simulink model "complete_model_sim_nolib"  (R2023b)
settings: Solver=VariableStepAuto  StartTime=0.0  StopTime=1e4  RelTol=1e-3
values from neighbouring files (symbols this model uses):
  a = 6.851221970532768e+03    (= 6851.22197053)    [complete_model.m]
  alpha1 = 0.4    [complete_model.m]
  alpha2 = 0.1    [complete_model.m]
  alpha3 = 0.5    [complete_model.m]
  D = zeros(3)    [complete_model.m]
  e = 0    [complete_model.m]
  FOV_earth = deg2rad(33)    [complete_model.m]
  FOV_sun = deg2rad(100)    [complete_model.m]
  freq_earth = 5    [complete_model.m]
  freq_mag = 5    [complete_model.m]
  freq_sun = 5    [complete_model.m]
  I = diag([I1 I2 I3])    [complete_model.m]    (also in compute_integral.m = I + (y(i + 1) + y(i) ) * (t(i + 1) - t(i)) * 0.5)
  Iinv = I\eye(3)    [complete_model.m]
  jb = [0.01; 0.05; 0.01]    [complete_model.m]
  k_gain = (4*pi/T) * (1 + sin(chsi)) * I2    [complete_model.m]
  mu = astroConstants(13)    [complete_model.m]
  n = sqrt(mu/a^3)    [complete_model.m]
  omega0 = 0.06 * rand(3,1)    [complete_model.m]
  omegaE = deg2rad(15)/3600    [complete_model.m]
  rs = -rr    [complete_model.m]
  s0 = 2*pi*rand(3,1)    [complete_model.m]
  tol = 0.2    [complete_model.m]
undefined symbols (not defined in the file or in its folder): gh, magnitude
libraries: cstextras x3, matrix_library x2, simulink_extras x1
(part 1 of 3)
settings Model: Creator=marcellopareschi  LastModifiedBy=turcu

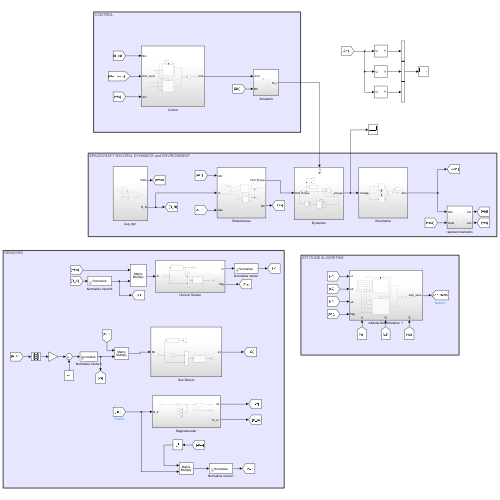
[thumbnail: Simulink's stored preview of the top-level diagram]
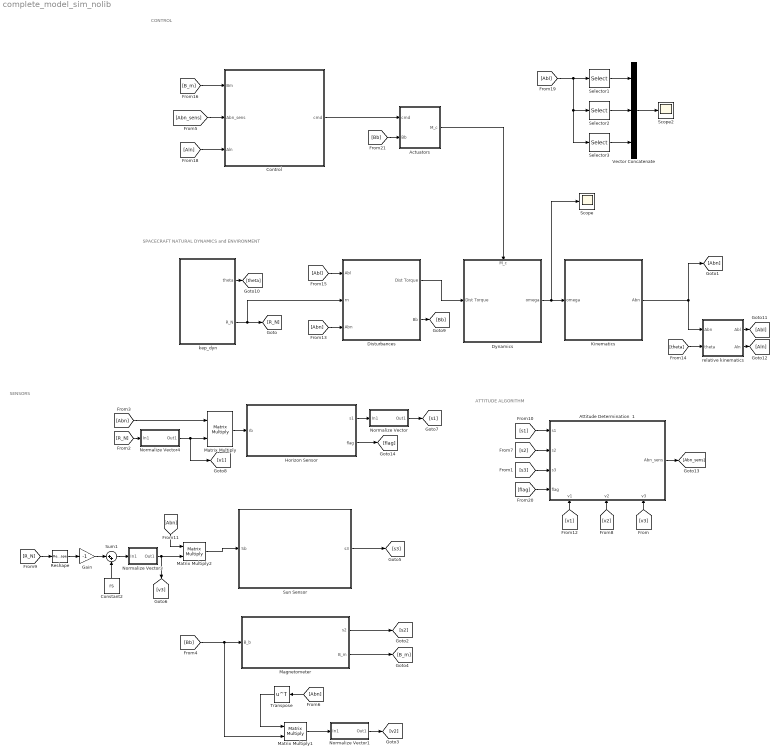
== system complete_model_sim_nolib ==
  note: SPACECRAFT NATURAL DYNAMICS and ENVIRONMENT
  note: CONTROL
  note: ATTITUDE ALGORITHM
  note: SENSORS
  " Actuators" : Subsystem
  Attitude Determination  1 : Subsystem
      settings: PortSchema="{\"entries\":[{\"content\":{\"sides\":[{\"content\":{\"connectorIds\":[\"In1\",\"In2\",\"In3\",\"In4\"]},\"type\":\"ConnectorPlacement.EquallySpacedRectSide\",\"uuid\":\"730966cf-d0d7-44a0-92f0-b5324480e7cc\"},{\"content\":{\"connectorIds\":[\"Out1\"],\"side\":\"RIGHT\"},\"type\":\"ConnectorPlacement.EquallySpacedRectSide\",\"uuid\":\"c83e6b57-46fe-4a45-9824-d3495e15bf6a\"},{\"content\":{\"side\":\"TOP\"},\"type\":\"ConnectorPlacement.EquallySpacedRectSide\",\"uuid\":\"4938c298-c2b3-45b7-bcb0-70b8132dabc6\"},{\"content\":{\"connectorIds\":[\"In5\",\"In6\",\"In7\"],\"side\":\"BOTTOM\"},\"type\":\"ConnectorPlacement.EquallySpacedRectSide\",\"uuid\":\"6d6a244e-80db-423b-a0a5-9a5face48fcb\"}]},\"type\":\"ConnectorPlacement.EquallySpacedConnector\",\"uuid\":\"7eb6767d-3ff0-4577-86c9-ebc5e763f220\"}],\"packageUris\":[\"http://schema.mathworks.com/mf0/Connector/R2020b\"],\"version\":\"1.0\"}"
  Constant2 : Constant  Value=rs
  Control : Subsystem
  Disturbances : Subsystem
  Dynamics : Subsystem
      settings: PortSchema="{\"entries\":[{\"content\":{\"sides\":[{\"content\":{\"connectorIds\":[\"In1\"]},\"type\":\"ConnectorPlacement.EquallySpacedRectSide\",\"uuid\":\"c50eaaef-bc5a-4b30-975a-dad3b72c53e1\"},{\"content\":{\"connectorIds\":[\"Out1\"],\"side\":\"RIGHT\"},\"type\":\"ConnectorPlacement.EquallySpacedRectSide\",\"uuid\":\"08d23e91-5daf-4f03-95f9-71d6696597c3\"},{\"content\":{\"connectorIds\":[\"In2\"],\"side\":\"TOP\"},\"type\":\"ConnectorPlacement.EquallySpacedRectSide\",\"uuid\":\"7ec65280-cc3e-44b1-8843-81c3a216d755\"}]},\"type\":\"ConnectorPlacement.EquallySpacedConnector\",\"uuid\":\"721d018a-ab6c-4a15-8dbf-409a72b03ba1\"}],\"packageUris\":[\"http://schema.mathworks.com/mf0/Connector/R2020b\"],\"version\":\"1.0\"}"
  Gain : Gain  Gain=-1
  Horizon Sensor : Subsystem
  Kinematics : Subsystem
  Magnetometer : Subsystem
  Matrix Multiply : Product  Multiplication=Matrix(*)
  Matrix Multiply1 : Product  Multiplication=Matrix(*)
  Matrix Multiply2 : Product  Multiplication=Matrix(*)
  Normalize Vector : Subsystem  mask(Normalize Vector){maxzero=0}
      mask prompts: maxzero "Maximum modulus to treat vector as zero:"
      mask help:
      | Normalize a vector.
      | Output is the unit vector parallel to the input vector. Input can be vector of any size.
      | If the modulus of the input is lower or equal than specified, the output is set to zeros(size(u)).
      settings: LibrarySourceBlock=vrlib/Utilities/Normalize Vector
      mask Help: helpview(vrmfunc('FnHelpTopic'), 'vr_normalizevector');
      mask Display: disp('Normalize')
  Normalize Vector1 : Subsystem  mask(Normalize Vector){maxzero=0}
      mask prompts: maxzero "Maximum modulus to treat vector as zero:"
      mask help:
      | Normalize a vector.
      | Output is the unit vector parallel to the input vector. Input can be vector of any size.
      | If the modulus of the input is lower or equal than specified, the output is set to zeros(size(u)).
      settings: LibrarySourceBlock=vrlib/Utilities/Normalize Vector
      mask Help: helpview(vrmfunc('FnHelpTopic'), 'vr_normalizevector');
      mask Display: disp('Normalize')
  Normalize Vector3 : Subsystem  mask(Normalize Vector){maxzero=0}
      mask prompts: maxzero "Maximum modulus to treat vector as zero:"
      mask help:
      | Normalize a vector.
      | Output is the unit vector parallel to the input vector. Input can be vector of any size.
      | If the modulus of the input is lower or equal than specified, the output is set to zeros(size(u)).
      settings: LibrarySourceBlock=vrlib/Utilities/Normalize Vector
      mask Help: helpview(vrmfunc('FnHelpTopic'), 'vr_normalizevector');
      mask Display: disp('Normalize')
  Normalize Vector4 : Subsystem  mask(Normalize Vector){maxzero=0}
      mask prompts: maxzero "Maximum modulus to treat vector as zero:"
      mask help:
      | Normalize a vector.
      | Output is the unit vector parallel to the input vector. Input can be vector of any size.
      | If the modulus of the input is lower or equal than specified, the output is set to zeros(size(u)).
      settings: LibrarySourceBlock=vrlib/Utilities/Normalize Vector
      mask Help: helpview(vrmfunc('FnHelpTopic'), 'vr_normalizevector');
      mask Display: disp('Normalize')
  Reshape : Reshape  OutputDimensionality=Column vector (2-D)
  Scope : Scope
  Scope2 : Scope
  Selector1 : Selector  NumberOfDimensions=2  InputPortWidth=3  IndexOptions=Index vector (dialog),Index vector (dialog)  Indices=3,2  OutputSizes=1,1
  Selector2 : Selector  NumberOfDimensions=2  InputPortWidth=3  IndexOptions=Index vector (dialog),Index vector (dialog)  Indices=1,3  OutputSizes=1,1
  Selector3 : Selector  NumberOfDimensions=2  InputPortWidth=3  IndexOptions=Index vector (dialog),Index vector (dialog)  Indices=2,1  OutputSizes=1,1
  Sum1 : Sum  Inputs=|++
  Sun Sensor : Subsystem
  Transpose : Math  Operator=transpose
  Vector Concatenate : Concatenate  NumInputs=3
  kep_dyn : Subsystem
  relative kinematics : Subsystem
  wires:
  Normalize Vector3/1(Out1) -> Matrix Multiply2/2, [v3]
  Magnetometer/1(s2) -> [s2]
  [Abn] -> Transpose/1
  Matrix Multiply1/1 -> Normalize Vector1/1(In1)
  Transpose/1 -> Matrix Multiply1/1
  [theta] -> relative kinematics/2(theta)
  [v1] -> Attitude Determination  1/5(v1)
  [Abn] -> Matrix Multiply/1
  [R_N] -> Reshape/1
  Gain/1 -> Sum1/1
  [Bb] -> Matrix Multiply1/2, Magnetometer/1(B_b)
  Normalize Vector4/1(Out1) -> [v1], Matrix Multiply/2
  [s3] -> Attitude Determination  1/3(s3)
  Normalize Vector1/1(Out1) -> [v2]
  " Actuators"/1(M_c) -> Dynamics/2(M_c)
  Magnetometer/2("B_m ") -> [B_m]
  Sun Sensor/1(s3) -> [s3]
  [R_N] -> Normalize Vector4/1(In1)
  Constant2/1 -> Sum1/2
  [s2] -> Attitude Determination  1/2(s2)
  Matrix Multiply/1 -> Horizon Sensor/1(rb)
  Reshape/1 -> Gain/1
  Normalize Vector/1(Out1) -> [s1]
  [v3] -> Attitude Determination  1/7(v3)
  [s1] -> Attitude Determination  1/1(s1)
  Sum1/1 -> Normalize Vector3/1(In1)
  Attitude Determination  1/1(Abn_sens) -> [Abn_sens]
  relative kinematics/1(Abl) -> [Abl]
  Kinematics/1(Abn) -> [Abn], relative kinematics/1(Abn)
  relative kinematics/2(Aln) -> [Aln]
  [Abn] -> Matrix Multiply2/1
  Dynamics/1(omega) -> Scope/1, Kinematics/1(omega)
  [v2] -> Attitude Determination  1/6(v2)
  Horizon Sensor/1(s1) -> Normalize Vector/1(In1)
  Matrix Multiply2/1 -> Sun Sensor/1(Sb)
  [Bb] -> " Actuators"/2(Bb)
  [B_m] -> Control/1(Bm)
  [Abn_sens] -> Control/2(Abn_sens)
  [Aln] -> Control/3(Aln)
  Control/1(cmd) -> " Actuators"/1(cmd)
  [Abl] -> Selector3/1, Selector2/1, Selector1/1
  Selector2/1 -> Vector Concatenate/2
  Selector3/1 -> Vector Concatenate/3
  Selector1/1 -> Vector Concatenate/1
  Vector Concatenate/1 -> Scope2/1
  Horizon Sensor/2(flag) -> [flag]
  [flag] -> Attitude Determination  1/4(flag)
  [Abl] -> Disturbances/1(Abl)
  kep_dyn/1(theta) -> [theta]
  [Abn] -> Disturbances/3(Abn)
  Disturbances/1(Dist Torque) -> Dynamics/1(Dist Torque)
  Disturbances/2(Bb) -> [Bb]
  kep_dyn/2(R_N) -> Disturbances/2(rn), [R_N]

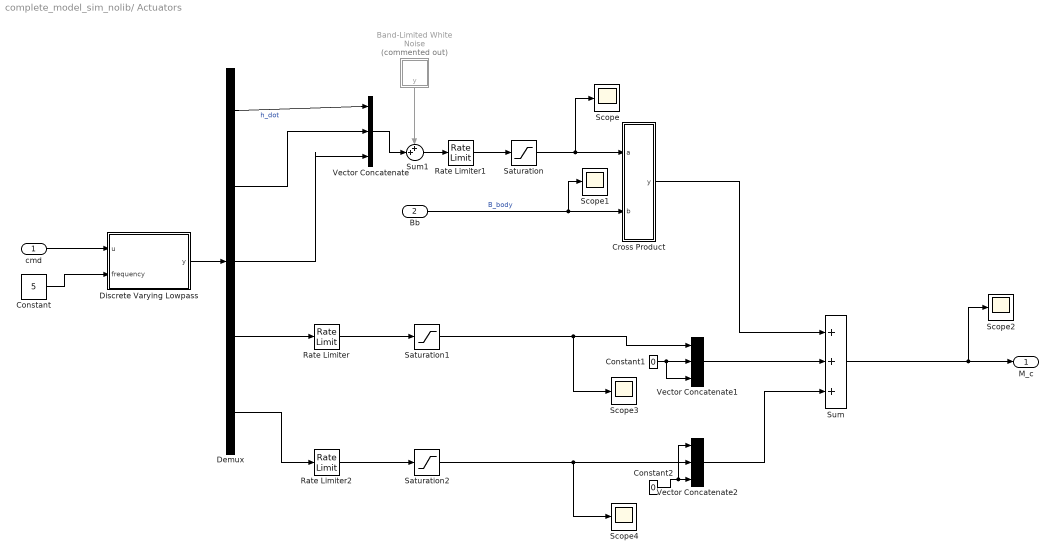
== system complete_model_sim_nolib/ Actuators ==
  cmd : Inport
  Bb : Inport  Port=2
  Band-Limited White Noise : Subsystem  Commented=on  mask(Band-Limited White Noise.){Cov=[0.1], Ts=1/30, seed=[23341], VectorParams1D=on}
      mask prompts: Cov "Simulink:masks:NoisePower_MP"; Ts "Simulink:masks:SampleTime_MP"; seed "Simulink:masks:Seed_MP"; VectorParams1D "Simulink:masks:InterpretVectorParametersAs1D_MP"
      mask help: Simulink:masks:BandLimitedWhiteNoise_MD
      mask init:
      | if any(Cov < 0),
      | 	error('The ''Noise power'' must be positive. '),
      | end;
      | 
      | r = [-0.4326
      |    -1.6656
      |     0.1253
      |     0.2877
      |    -1.1465
      |     1.1909
      |     1.1892
      |    -0.0376
      |     0.3273
      |     0.1746
      |    -0.1867
      |     0.7258]';
      | 
      | r2 = [r(1),r;r,r(12)]; 
      | t =[1:13;1:13]; 
      | 
      | if any(Ts==-1), 
      | 	error('Sample time (-1) is set to be back-inherited from the block(s) it drives. You should explicitly specify the sample time of the source block. '), 
      | end;
      | 
      | if ~isdeployed
      | set_param([gcb '/White Noise'],'VectorParams1D',VectorParams1D);
      | end
      settings: LibrarySourceBlock=|
      | simulink/Sources/Band-Limited
      | White Noise
      mask Help: Implemented using white noise into Zero-Order Hold block. The seed and power can be vectors of the same length to produce a vector of white noise sources. For faster simulation, set sample time to the highest value possible but in accordance with the fastest dynamics of system.
  Constant : Constant  Value=5
  Constant1 : Constant  Value=0
  Constant2 : Constant  Value=0
  Cross Product : Subsystem  mask(CrossProduct){}
      mask help: Simulink:masks:MatLibCrossProduct_MD
      settings: LibrarySourceBlock=|
      | simulink/Matrix
      | Operations/Cross Product
      mask Display: disp('cross')
  Demux : Demux  Outputs=5
  Discrete Varying Lowpass : Subsystem  mask(Discrete Varying Lowpass){N=2, w0=0, Ts=1/30}
      mask prompts: N "Control:simulink:VaryingLowpassLabel1"; w0 "Control:simulink:VaryingLowpassLabel2"; Ts "Control:simulink:VaryingLowpassLabel3"
      mask help: Control:simulink:VaryingLowpass2
      mask init:
      | if N~=round(N)
      |    hCB = get_param(gcb,'handle');
      |    DAStudio.slerror('Control:simulink:InvalidOrder',hCB)
      | elseif w0*Ts>=pi
      |    hCB = get_param(gcb,'handle');
      |    DAStudio.slerror('Control:simulink:InvalidPrewarp',hCB)
      | end
      | SimStatus = get_param(bdroot,'SimulationStatus');
      | if any(strcmp(SimStatus,{'initializing','updating','stopped'}))
      |    controllib.internal.blocks.varying.varyingLP(gcb,N,Ts)
      | end
      settings: LibrarySourceBlock=cstblocks/Linear Parameter Varying/Discrete Varying Lowpass
      mask Help: eval('helpview(''control'',''VaryingLowpassDT'');')
      mask DialogControl N Prompt: Filter order:
      mask DialogControl w0 Prompt: Pre-warping frequency w0 (rad/s):
      mask DialogControl Ts Prompt: Sample time Ts:
      mask Display:
      | image('lowpass_dt.png',[0.1 0 0.8 1]);
      | port_label('input', 2, 'freq');
  Rate Limiter : RateLimiter
  Rate Limiter1 : RateLimiter  RisingSlewLimit=10  FallingSlewLimit=-10
  Rate Limiter2 : RateLimiter
  Saturation : Saturate  UpperLimit=150  LowerLimit=-150
  Saturation1 : Saturate
  Saturation2 : Saturate
  Scope{,1..4} (5 alike) : Scope
  Sum : Sum  Inputs=+++
  Sum1 : Sum  Inputs=++|
  Vector Concatenate : Concatenate  NumInputs=3
  Vector Concatenate1 : Concatenate  NumInputs=3
  Vector Concatenate2 : Concatenate  NumInputs=3
  M_c : Outport
  wires:
  Bb/1 -> Scope1/1, Cross Product/2(b)  "B_body"
  Rate Limiter1/1 -> Saturation/1
  Band-Limited White Noise/1(y) -> Sum1/1
  Sum1/1 -> Rate Limiter1/1
  Saturation/1 -> Scope/1, Cross Product/1(a)
  Vector Concatenate/1 -> Sum1/2
  Constant1/1 -> Vector Concatenate1/3, Vector Concatenate1/2
  Sum/1 -> Scope2/1, M_c/1
  Rate Limiter/1 -> Saturation1/1
  Saturation1/1 -> Scope3/1, Vector Concatenate1/1
  Demux/1 -> Vector Concatenate/1  "h_dot"
  Demux/2 -> Vector Concatenate/2
  Demux/3 -> Vector Concatenate/3
  Demux/4 -> Rate Limiter/1
  Saturation2/1 -> Vector Concatenate2/2, Scope4/1
  Constant2/1 -> Vector Concatenate2/1, Vector Concatenate2/3
  Rate Limiter2/1 -> Saturation2/1
  Demux/5 -> Rate Limiter2/1
  Vector Concatenate1/1 -> Sum/2
  Cross Product/1(y) -> Sum/1
  Vector Concatenate2/1 -> Sum/3
  Constant/1 -> Discrete Varying Lowpass/2(frequency)
  Discrete Varying Lowpass/1(y) -> Demux/1
  cmd/1 -> Discrete Varying Lowpass/1(u)

== system complete_model_sim_nolib/Attitude Determination  1 ==
  s1 : Inport
  s2 : Inport  Port=2
  s3 : Inport  Port=3
  flag : Inport  Port=4
  v1 : Inport  Port=5
  v2 : Inport  Port=6
  v3 : Inport  Port=7
  Enabled Subsystem : Subsystem  TreatAsAtomicUnit=on
  Merge : Merge
  NOT : Logic  Operator=NOT  IconShape=distinctive  AllPortsSameDT=off  OutDataTypeStr=boolean
  Statistical Method : Subsystem  TreatAsAtomicUnit=on
  Abn_sens : Outport
  wires:
  flag/1 -> NOT/1, Statistical Method/Enable
  s1/1 -> Statistical Method/1(s1)
  s2/1 -> Enabled Subsystem/1(q), Statistical Method/2(s2)
  s3/1 -> Enabled Subsystem/2(p), Statistical Method/3(s3)
  v1/1 -> Statistical Method/4(v1)
  v2/1 -> Enabled Subsystem/3(b), Statistical Method/5(v2)
  v3/1 -> Enabled Subsystem/4(a), Statistical Method/6(v3)
  NOT/1 -> Enabled Subsystem/Enable
  Statistical Method/1(Abn_sens) -> Merge/1
  Enabled Subsystem/1(A_bn_sens) -> Merge/2
  Merge/1 -> Abn_sens/1

== system complete_model_sim_nolib/Control ==
  Bm : Inport
  Abn_sens : Inport  Port=2
  Aln : Inport  Port=3
  De-Tumbling Bdot control1 : Subsystem
  Merge : Merge
  NOT : Logic  Operator=NOT  IconShape=distinctive  AllPortsSameDT=off  OutDataTypeStr=boolean
  Scope1 : Scope
  Slew Maneuver : Subsystem
  Unit Delay : UnitDelay  InitialCondition=1  SampleTime=-1  HasFrameUpgradeWarning=on
  cmd : Outport
  wires:
  Unit Delay/1 -> NOT/1, Scope1/1, De-Tumbling Bdot control1/Enable
  De-Tumbling Bdot control1/2(flag) -> Unit Delay/1
  Bm/1 -> Slew Maneuver/3(B_m), De-Tumbling Bdot control1/1(B_m)
  Abn_sens/1 -> Slew Maneuver/1(Abn_sens)
  Aln/1 -> Slew Maneuver/2(Aln)
  NOT/1 -> Slew Maneuver/Enable
  Slew Maneuver/1(cmd) -> Merge/2
  De-Tumbling Bdot control1/1(cmd) -> Merge/1
  Merge/1 -> cmd/1

== system complete_model_sim_nolib/Disturbances ==
  Abl : Inport
  rn : Inport  Port=2
  Abn : Inport  Port=3
  Constant : Constant  Value=[1; 0; 0]
  "Magnetic Torque " : Subsystem
  Matrix Multiply : Product  Multiplication=Matrix(*)
  Scope1 : Scope
  Sum : Sum  Inputs=|++
  To Workspace : ToWorkspace  VariableName=GG_torque  SampleTime=-1
  To Workspace1 : ToWorkspace  VariableName=mag_torque  SampleTime=-1
  gravity torque : Subsystem
  norm : Subsystem
  Dist Torque : Outport
  Bb : Outport  Port=2
  wires:
  Abl/1 -> Matrix Multiply/1
  Constant/1 -> Matrix Multiply/2
  Matrix Multiply/1 -> gravity torque/1(c)
  rn/1 -> norm/1(rn), "Magnetic Torque "/1(rn)
  Abn/1 -> "Magnetic Torque "/2(Abn)
  gravity torque/1(Mg) -> To Workspace/1, Sum/1
  "Magnetic Torque "/1(M_mag) -> To Workspace1/1, Sum/2, Scope1/1
  Sum/1 -> Dist Torque/1
  "Magnetic Torque "/2(Bb) -> Bb/1
  norm/1(rnorm) -> gravity torque/2(rnorm)

== system complete_model_sim_nolib/Dynamics ==
  Dist Torque : Inport
  M_c : Inport  Port=2
  Constant : Constant  Value=I
  Constant1 : Constant  Value=Iinv
  Cross Product : Subsystem  mask(CrossProduct){}
      mask help: Simulink:masks:MatLibCrossProduct_MD
      settings: LibrarySourceBlock=|
      | simulink/Matrix
      | Operations/Cross Product
      mask Display: disp('cross')
  Integrator : Integrator  InitialCondition=omega0
  Product : Product  Multiplication=Matrix(*)
  Product1 : Product  Multiplication=Matrix(*)
  Scope : Scope
  Scope1 : Scope
  Sum : Sum  Inputs=+++
  To Workspace : ToWorkspace  VariableName=omegab  SampleTime=-1
  omega : Outport
  wires:
  Constant/1 -> Product/1
  Product1/1 -> Integrator/1
  Integrator/1 -> omega/1, Scope/1, To Workspace/1, Cross Product/2(b), Product/2
  Product/1 -> Cross Product/1(a)
  Constant1/1 -> Product1/1
  Cross Product/1(y) -> Sum/2
  Sum/1 -> Product1/2
  Dist Torque/1 -> Sum/3
  M_c/1 -> Scope1/1, Sum/1

== system complete_model_sim_nolib/Horizon Sensor ==
  rb : Inport
  EH sensor modeling : Subsystem
  FOV CHECK : Subsystem
  Product1 : Product
  s1 : Outport
  flag : Outport  Port=2
  wires:
  rb/1 -> FOV CHECK/1(rb), Product1/2
  Product1/1 -> EH sensor modeling/1(rb)
  EH sensor modeling/1(q) -> s1/1  "direction of earth"
  FOV CHECK/1(b) -> Product1/1, flag/1

== system complete_model_sim_nolib/Kinematics ==
  omega : Inport
  Kinematics 312 : Subsystem
  Kinematics 313 : Subsystem
  Merge : Merge
  NOT : Logic  Operator=NOT  IconShape=distinctive  AllPortsSameDT=off  OutDataTypeStr=boolean
  System switcher : Subsystem
  To Workspace : ToWorkspace  VariableName=A  SaveFormat=Timeseries  SampleTime=-1
  Abn : Outport
  wires:
  NOT/1 -> Kinematics 313/Enable
  omega/1 -> Kinematics 312/1(w), Kinematics 313/1(w)
  System switcher/1(flag) -> Kinematics 312/Enable, NOT/1
  Kinematics 313/1(A) -> Merge/2
  Merge/1 -> Abn/1, To Workspace/1  "A"
  Kinematics 312/1(A) -> Merge/1

== system complete_model_sim_nolib/Magnetometer ==
  B_b : Inport
  Band-Limited White Noise : Subsystem  mask(Band-Limited White Noise.){Cov=[1.18^2 *1e-18], Ts=1/30, seed=[23341], VectorParams1D=on}
      mask prompts: Cov "Simulink:masks:NoisePower_MP"; Ts "Simulink:masks:SampleTime_MP"; seed "Simulink:masks:Seed_MP"; VectorParams1D "Simulink:masks:InterpretVectorParametersAs1D_MP"
      mask help: Simulink:masks:BandLimitedWhiteNoise_MD
      mask init: same as complete_model_sim_nolib/ Actuators/Band-Limited White Noise
      settings: LibrarySourceBlock=|
      | simulink/Sources/Band-Limited
      | White Noise
      mask Help: Implemented using white noise into Zero-Order Hold block. The seed and power can be vectors of the same length to produce a vector of white noise sources. For faster simulation, set sample time to the highest value possible but in accordance with the fastest dynamics of system.
  Band-Limited White Noise1 : Subsystem  mask(Band-Limited White Noise.){Cov=[1.18^2 *1e-18], Ts=1/30, seed=[23341], VectorParams1D=on}
      mask prompts: Cov "Simulink:masks:NoisePower_MP"; Ts "Simulink:masks:SampleTime_MP"; seed "Simulink:masks:Seed_MP"; VectorParams1D "Simulink:masks:InterpretVectorParametersAs1D_MP"
      mask help: Simulink:masks:BandLimitedWhiteNoise_MD
      mask init: same as complete_model_sim_nolib/ Actuators/Band-Limited White Noise
      settings: LibrarySourceBlock=|
      | simulink/Sources/Band-Limited
      | White Noise
      mask Help: Implemented using white noise into Zero-Order Hold block. The seed and power can be vectors of the same length to produce a vector of white noise sources. For faster simulation, set sample time to the highest value possible but in accordance with the fastest dynamics of system.
  Band-Limited White Noise2 : Subsystem  mask(Band-Limited White Noise.){Cov=[1.18^2 *1e-18], Ts=1/30, seed=[23341], VectorParams1D=on}
      mask prompts: Cov "Simulink:masks:NoisePower_MP"; Ts "Simulink:masks:SampleTime_MP"; seed "Simulink:masks:Seed_MP"; VectorParams1D "Simulink:masks:InterpretVectorParametersAs1D_MP"
      mask help: Simulink:masks:BandLimitedWhiteNoise_MD
      mask init: same as complete_model_sim_nolib/ Actuators/Band-Limited White Noise
      settings: LibrarySourceBlock=|
      | simulink/Sources/Band-Limited
      | White Noise
      mask Help: Implemented using white noise into Zero-Order Hold block. The seed and power can be vectors of the same length to produce a vector of white noise sources. For faster simulation, set sample time to the highest value possible but in accordance with the fastest dynamics of system.
  Normalize Vector : Subsystem  mask(Normalize Vector){maxzero=0}
      mask prompts: maxzero "Maximum modulus to treat vector as zero:"
      mask help:
      | Normalize a vector.
      | Output is the unit vector parallel to the input vector. Input can be vector of any size.
      | If the modulus of the input is lower or equal than specified, the output is set to zeros(size(u)).
      settings: LibrarySourceBlock=vrlib/Utilities/Normalize Vector
      mask Help: helpview(vrmfunc('FnHelpTopic'), 'vr_normalizevector');
      mask Display: disp('Normalize')
  Sum : Sum  Inputs=|++
  Vector Concatenate1 : Concatenate  NumInputs=3
  Zero-Order Hold2 : ZeroOrderHold  SampleTime=1/freq_mag
  s2 : Outport
  "B_m " : Outport  Port=2
  wires:
  Zero-Order Hold2/1 -> Sum/1  "B_B"
  Band-Limited White Noise2/1(y) -> Vector Concatenate1/3
  Band-Limited White Noise1/1(y) -> Vector Concatenate1/2
  Band-Limited White Noise/1(y) -> Vector Concatenate1/1
  Normalize Vector/1(Out1) -> s2/1
  Vector Concatenate1/1 -> Sum/2
  Sum/1 -> "B_m "/1, Normalize Vector/1(In1)
  B_b/1 -> Zero-Order Hold2/1  "B_B"

== system complete_model_sim_nolib/Normalize Vector ==
  In1 : Inport
  Constant : Constant
  Demux : Demux  Outputs=[-1 1]
  Divide : Product  Inputs=*/  OutDataTypeStr=double
  Ground : Ground
  Math Function : Math  Operator=square  SignedPower=on
  Math Function1 : Math  Operator=sqrt  SignedPower=on
  Mux : Mux  Inputs=2
  Mux1 : Mux  Inputs=2
  Product : Product  RndMeth=Zero
  Sum of Elements : Sum  Inputs=+
  Switch : Switch  Criteria=u2 > Threshold  Threshold=maxzero  SaturateOnIntegerOverflow=off  InputSameDT=off
  Out1 : Outport  VectorParamsAs1DForOutWhenUnconnected=off
  wires:
  Ground/1 -> Product/2
  Product/1 -> Mux1/1
  Constant/1 -> Mux1/2
  Mux1/1 -> Switch/3
  Sum of Elements/1 -> Math Function1/1
  Math Function/1 -> Sum of Elements/1
  Demux/2 -> Divide/2
  Demux/1 -> Divide/1
  Switch/1 -> Demux/1
  Mux/1 -> Switch/1
  Math Function1/1 -> Mux/2, Switch/2
  In1/1 -> Product/1, Math Function/1, Mux/1
  Divide/1 -> Out1/1

== system complete_model_sim_nolib/Normalize Vector1 ==
  In1 : Inport
  Constant : Constant
  Demux : Demux  Outputs=[-1 1]
  Divide : Product  Inputs=*/  OutDataTypeStr=double
  Ground : Ground
  Math Function : Math  Operator=square  SignedPower=on
  Math Function1 : Math  Operator=sqrt  SignedPower=on
  Mux : Mux  Inputs=2
  Mux1 : Mux  Inputs=2
  Product : Product  RndMeth=Zero
  Sum of Elements : Sum  Inputs=+
  Switch : Switch  Criteria=u2 > Threshold  Threshold=maxzero  SaturateOnIntegerOverflow=off  InputSameDT=off
  Out1 : Outport  VectorParamsAs1DForOutWhenUnconnected=off
  wires:
  Ground/1 -> Product/2
  Product/1 -> Mux1/1
  Constant/1 -> Mux1/2
  Mux1/1 -> Switch/3
  Sum of Elements/1 -> Math Function1/1
  Math Function/1 -> Sum of Elements/1
  Demux/2 -> Divide/2
  Demux/1 -> Divide/1
  Switch/1 -> Demux/1
  Mux/1 -> Switch/1
  Math Function1/1 -> Mux/2, Switch/2
  In1/1 -> Product/1, Math Function/1, Mux/1
  Divide/1 -> Out1/1

== system complete_model_sim_nolib/Normalize Vector3 ==
  In1 : Inport
  Constant : Constant
  Demux : Demux  Outputs=[-1 1]
  Divide : Product  Inputs=*/  OutDataTypeStr=double
  Ground : Ground
  Math Function : Math  Operator=square  SignedPower=on
  Math Function1 : Math  Operator=sqrt  SignedPower=on
  Mux : Mux  Inputs=2
  Mux1 : Mux  Inputs=2
  Product : Product  RndMeth=Zero
  Sum of Elements : Sum  Inputs=+
  Switch : Switch  Criteria=u2 > Threshold  Threshold=maxzero  SaturateOnIntegerOverflow=off  InputSameDT=off
  Out1 : Outport  VectorParamsAs1DForOutWhenUnconnected=off
  wires:
  Ground/1 -> Product/2
  Product/1 -> Mux1/1
  Constant/1 -> Mux1/2
  Mux1/1 -> Switch/3
  Sum of Elements/1 -> Math Function1/1
  Math Function/1 -> Sum of Elements/1
  Demux/2 -> Divide/2
  Demux/1 -> Divide/1
  Switch/1 -> Demux/1
  Mux/1 -> Switch/1
  Math Function1/1 -> Mux/2, Switch/2
  In1/1 -> Product/1, Math Function/1, Mux/1
  Divide/1 -> Out1/1

== system complete_model_sim_nolib/Normalize Vector4 ==
  In1 : Inport
  Constant : Constant
  Demux : Demux  Outputs=[-1 1]
  Divide : Product  Inputs=*/  OutDataTypeStr=double
  Ground : Ground
  Math Function : Math  Operator=square  SignedPower=on
  Math Function1 : Math  Operator=sqrt  SignedPower=on
  Mux : Mux  Inputs=2
  Mux1 : Mux  Inputs=2
  Product : Product  RndMeth=Zero
  Sum of Elements : Sum  Inputs=+
  Switch : Switch  Criteria=u2 > Threshold  Threshold=maxzero  SaturateOnIntegerOverflow=off  InputSameDT=off
  Out1 : Outport  VectorParamsAs1DForOutWhenUnconnected=off
  wires:
  Ground/1 -> Product/2
  Product/1 -> Mux1/1
  Constant/1 -> Mux1/2
  Mux1/1 -> Switch/3
  Sum of Elements/1 -> Math Function1/1
  Math Function/1 -> Sum of Elements/1
  Demux/2 -> Divide/2
  Demux/1 -> Divide/1
  Switch/1 -> Demux/1
  Mux/1 -> Switch/1
  Math Function1/1 -> Mux/2, Switch/2
  In1/1 -> Product/1, Math Function/1, Mux/1
  Divide/1 -> Out1/1

== system complete_model_sim_nolib/Sun Sensor ==
  Sb : Inport
  Constant : Constant
  FOV CHECK : Subsystem
  Product : Product
  Scope : Scope
  Sun Sensor Modeling : Subsystem
  s3 : Outport
  wires:
  Sb/1 -> Product/2, FOV CHECK/1(In1)  "Sb"
  Sun Sensor Modeling/1(s3) -> s3/1
  Product/1 -> Sun Sensor Modeling/1(Sb)  "Sb"
  Constant/1 -> Product/1
  FOV CHECK/1(b) -> Scope/1

== system complete_model_sim_nolib/kep_dyn ==
  A_np : Constant  Value=A_pn'
  Constant : Constant  Value=0
  Constant1 : Constant  Value=e
  Cos : Trigonometry  Operator=cos
  Integrator : Integrator
  Matrix Multiply : Product  Multiplication=Matrix(*)
  Product2 : Product
  Sin : Trigonometry
  Vector Concatenate : Concatenate  NumInputs=3
  r_norm : Subsystem
  theta integration : Subsystem
      settings: PortSchema="{\"entries\":[{\"content\":{\"sides\":[{\"content\":{\"connectorIds\":[\"In1\"]},\"type\":\"ConnectorPlacement.EquallySpacedRectSide\",\"uuid\":\"3f1b1ec9-07ed-4eb1-9e41-630dc5613e97\"},{\"content\":{\"connectorIds\":[\"Out1\",\"In2\"],\"side\":\"RIGHT\"},\"type\":\"ConnectorPlacement.EquallySpacedRectSide\",\"uuid\":\"22d0f7bc-714c-4365-a26c-07047ff4be14\"},{\"content\":{\"side\":\"TOP\"},\"type\":\"ConnectorPlacement.EquallySpacedRectSide\",\"uuid\":\"875f7006-d698-4730-93ae-1a7d05f24054\"}]},\"type\":\"ConnectorPlacement.EquallySpacedConnector\",\"uuid\":\"799b65b1-faea-432b-9f3f-2d21984184cd\"}],\"packageUris\":[\"http://schema.mathworks.com/mf0/Connector/R2020b\"],\"version\":\"1.0\"}"
  theta : Outport
  R_N : Outport  Port=2
  wires:
  Integrator/1 -> r_norm/2(theta), theta/1, Sin/1, Cos/1, theta integration/1(theta)
  theta integration/1(theta_dot) -> Integrator/1
  Constant/1 -> Vector Concatenate/3
  Cos/1 -> Vector Concatenate/1
  Constant1/1 -> theta integration/2(e), r_norm/1(e)
  r_norm/1(r) -> Product2/1
  Vector Concatenate/1 -> Product2/2
  Sin/1 -> Vector Concatenate/2
  A_np/1 -> Matrix Multiply/1
  Product2/1 -> Matrix Multiply/2
  Matrix Multiply/1 -> R_N/1

== system complete_model_sim_nolib/relative kinematics ==
  Abn : Inport
  theta : Inport  Port=2
  Constant : Constant  Value=A_pn'
  Matrix Multiply : Product  Multiplication=Matrix(*)
  Matrix Multiply2 : Product  Multiplication=Matrix(*)
  Subsystem : Subsystem
  Transpose : Math  Operator=transpose
  Abl : Outport
  Aln : Outport  Port=2
  wires:
  Abn/1 -> Matrix Multiply2/1
  Matrix Multiply/1 -> Transpose/1, Matrix Multiply2/2  "A_nl"
  Matrix Multiply2/1 -> Abl/1
  theta/1 -> Subsystem/1(theta)
  Subsystem/1(A_PL) -> Matrix Multiply/2  "A_PL"
  Constant/1 -> Matrix Multiply/1  "A_np"
  Transpose/1 -> Aln/1

== system complete_model_sim_nolib/ Actuators/Band-Limited White Noise ==
  Output : Gain  Gain=sqrt(Cov)/sqrt(Ts(1))  SaturateOnIntegerOverflow=on  OutDataTypeStr=Inherit: Same as input  ParamDataTypeStr=Inherit: Same as input
  White Noise : RandomNumber  DisableCoverage=on  Seed=seed  SampleTime=Ts
  y : Outport
  wires:
  Output/1 -> y/1
  White Noise/1 -> Output/1

== system complete_model_sim_nolib/ Actuators/Cross Product ==
  note: Cross product of two 3x1 vectors a=[a1 a2 a3], b=[b1 b2 b3]:
      | y = a x b = (a2b3-a3b2)i + (a3b1-a1b3)j + (a1b2-a2b1)k
  a : Inport
  b : Inport  Port=2
  Element Product : Product  RndMeth=Simplest
  Selector2 : Selector  InputPortWidth=6  IndexOptions=Index vector (dialog)  Indices=[1 2 3]  OutputSizes=1
  Selector3 : Selector  InputPortWidth=6  IndexOptions=Index vector (dialog)  Indices=[4 5 6]  OutputSizes=1
  Sum : Sum  Inputs=+|-  RndMeth=Simplest
  a elements : Selector  InputPortWidth=3  IndexOptions=Index vector (dialog)  Indices=[2 3 1 3 1 2]  OutputSizes=1
  b elements : Selector  InputPortWidth=3  IndexOptions=Index vector (dialog)  Indices=[3 1 2 2 3 1]  OutputSizes=1
  y : Outport
  wires:
  Selector3/1 -> Sum/2
  Selector2/1 -> Sum/1
  Element Product/1 -> Selector2/1, Selector3/1
  b/1 -> b elements/1
  b elements/1 -> Element Product/2
  a elements/1 -> Element Product/1
  Sum/1 -> y/1
  a/1 -> a elements/1

== system complete_model_sim_nolib/ Actuators/Discrete Varying Lowpass ==
  u : Inport
  frequency : Inport  Port=2
  SOS1 : cstextras/DiscreteSecondOrderSection  VariantControl=order2  zeta=sin(1*pi/4)  Ts=Ts  w0=w0
  y : Outport  VectorParamsAs1DForOutWhenUnconnected=off
  wires:
  u/1 -> SOS1/1
  frequency/1 -> SOS1/2
  SOS1/1 -> y/1

== system complete_model_sim_nolib/Attitude Determination  1/Enabled Subsystem ==
  q : Inport
  p : Inport  Port=2
  b : Inport  Port=3
  a : Inport  Port=4
  Enable : EnablePort
  Matrix Multiply : Product  Multiplication=Matrix(*)
  S : Subsystem
  Transpose : Math  Operator=transpose
  V : Subsystem
  A_bn_sens : Outport
  wires:
  V/1(V) -> Transpose/1
  S/1(S) -> Matrix Multiply/1
  Transpose/1 -> Matrix Multiply/2
  Matrix Multiply/1 -> A_bn_sens/1
  q/1 -> S/1(q)
  p/1 -> S/2(p)
  b/1 -> V/1(b)
  a/1 -> V/2(a)

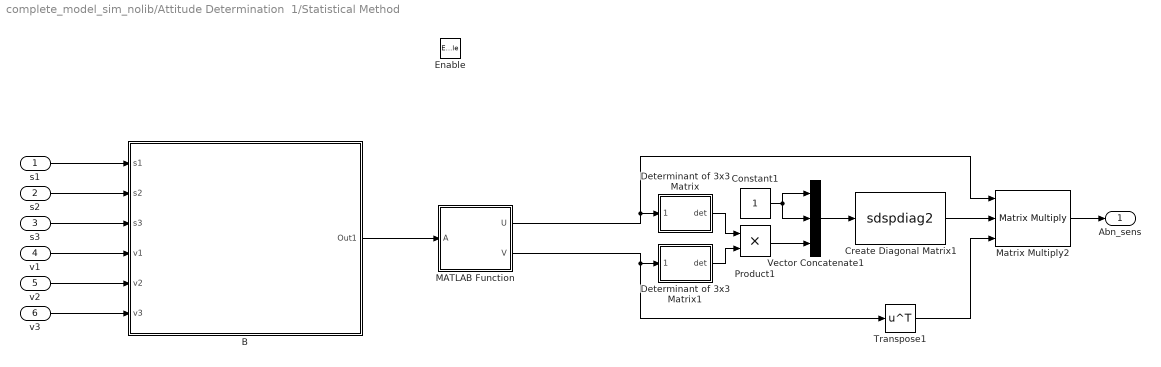
== system complete_model_sim_nolib/Attitude Determination  1/Statistical Method ==
  s1 : Inport
  s2 : Inport  Port=2
  s3 : Inport  Port=3
  v1 : Inport  Port=4
  v2 : Inport  Port=5
  v3 : Inport  Port=6
  Enable : EnablePort
  B : Subsystem
  Constant1 : Constant
  Create Diagonal Matrix1 : S-Function  FunctionName=sdspdiag2  Parameters=mode  SFunctionDeploymentMode=off  EnableBusSupport=off  mask(Create Diagonal Matrix){}
      mask help: Simulink:masks:CreateDiagonalMatrix_MD
      mask init:
      | mode = 1;
      settings: LibrarySourceBlock=|
      | simulink/Matrix
      | Operations/Create Diagonal
      | Matrix
      mask Display:
      | x = [.58 .87 .87 .58 .58 NaN 0.45 0.12 NaN 0.525 0.525 0.475 0.475 0.525 0.525 0.565 0.525 ];
      | y = [ 0.2 0.2 0.8 0.8 0.2 NaN 0.2 0.8 NaN 0.435 0.475 0.475 0.525 0.525 0.565 0.5 0.435 ];
      | plot(x,y);
      | port_label('input',1,'D');
      | port_label('output',1,'A');
  Determinant of 3x3 Matrix : Subsystem
      settings: LibrarySourceBlock=|
      | aerolibutil/Determinant of
      | 3x3 Matrix
  Determinant of 3x3 Matrix1 : Subsystem
      settings: LibrarySourceBlock=|
      | aerolibutil/Determinant of
      | 3x3 Matrix
  MATLAB Function : MATLAB Function  TreatAsAtomicUnit=on
  Matrix Multiply2 : Product  Inputs=3  Multiplication=Matrix(*)
  Product1 : Product
  Transpose1 : Math  Operator=transpose
  Vector Concatenate1 : Concatenate  NumInputs=3
  Abn_sens : Outport
  wires:
  MATLAB Function/2(V) -> Determinant of 3x3 Matrix1/1(Matrix), Transpose1/1
  MATLAB Function/1(U) -> Determinant of 3x3 Matrix/1(Matrix), Matrix Multiply2/1
  Vector Concatenate1/1 -> Create Diagonal Matrix1/1
  Transpose1/1 -> Matrix Multiply2/3
  Determinant of 3x3 Matrix1/1(det) -> Product1/2
  Product1/1 -> Vector Concatenate1/3
  Create Diagonal Matrix1/1 -> Matrix Multiply2/2
  Constant1/1 -> Vector Concatenate1/2, Vector Concatenate1/1
  Determinant of 3x3 Matrix/1(det) -> Product1/1
  B/1(Out1) -> MATLAB Function/1(A)
  s1/1 -> B/1(s1)
  s2/1 -> B/2(s2)
  s3/1 -> B/3(s3)
  v1/1 -> B/4(v1)
  v2/1 -> B/5(v2)
  v3/1 -> B/6(v3)
  Matrix Multiply2/1 -> Abn_sens/1

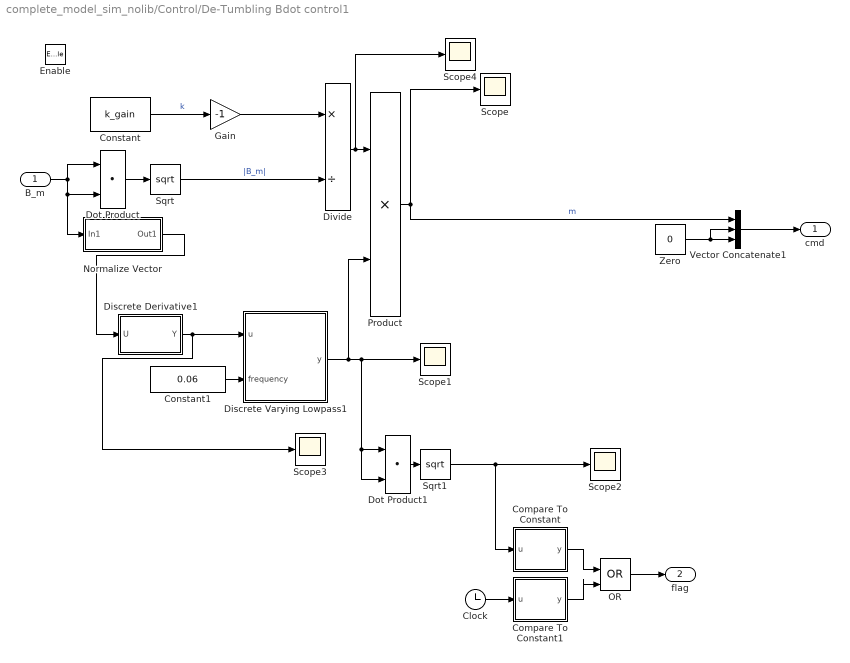
== system complete_model_sim_nolib/Control/De-Tumbling Bdot control1 ==
  B_m : Inport
  Enable : EnablePort
  Clock : Clock
  Compare To Constant : Subsystem  mask(Compare To Constant){relop=>=, const=0.003, OutDataTypeStr=boolean, ZeroCross=on}
      mask prompts: relop "Simulink:masks:Operator_MP"; const "Simulink:masks:ConstantValue_MP"; OutDataTypeStr "Simulink:masks:OutputDataType_MP"; ZeroCross "Simulink:masks:EnableZerocrossingDetection_MP"
      mask help: Simulink:masks:CompareToConstant_MD
      mask init:
      | blkName = gcb;
      | 
      | if strcmp(get_param(gcbh,'OutDataTypeStr'),'boolean')
      | 	setValue = 'boolean';
      | else
      | 	setValue = 'fixdt(0, 8, 0)';
      | end
      | 
      | set_param([blkName,'/Compare'],'relop',relop, ...
      | 	'OutDataTypeStr', setValue, 'ZeroCross', ZeroCross);
      | 
      | str = [relop,' C']; %default
      | 
      | const_str = get_param(blkName, 'const');
      | const_val = str2num(const_str);
      | 
      | if isempty(const_val) %#ok<ST2NM>
      |     %Expression/Variable
      |     str = [relop, ' ', strtrim(const_str)];
      | else
      |     if length(const_val) == 1 
      |         if Simulink.data.isSupportedEnumClass(class(const_val))
      |             % Special Handling for Enumerations
      |             if Simulink.data.getEnumTypeInfo(class(const_val), 'AddClassNameToEnumNames')
      |                 str = [relop, ' ', strtrim(const_str)];
      |             else
      |                 str = [relop, ' ', char(const_val)];
      |             end
      |         elseif(isfloat(const_val) || isinteger(const_val) || islogical(const_val)) 
      |                 str = [relop, ' ', num2str(const_val)];
      |         end
      |     end
      | end
      settings: LibrarySourceBlock=|
      | simulink/Logic and Bit
      | Operations/Compare
      | To Constant
      mask TypeOptions relop: == | ~= | < | <= | >= | >
      mask TypeOptions OutDataTypeStr: Simulink:masks:uint8 | Simulink:masks:boolean
      mask Callback ZeroCross: sl('zeroCrossEnable', gcbh);
      mask Display: disp(str)
  Compare To Constant1 : Subsystem  mask(Compare To Constant){relop=<=, const=10, OutDataTypeStr=boolean, ZeroCross=on}
      mask prompts: relop "Simulink:masks:Operator_MP"; const "Simulink:masks:ConstantValue_MP"; OutDataTypeStr "Simulink:masks:OutputDataType_MP"; ZeroCross "Simulink:masks:EnableZerocrossingDetection_MP"
      mask help: Simulink:masks:CompareToConstant_MD
      mask init: same as complete_model_sim_nolib/Control/De-Tumbling Bdot control1/Compare To Constant
      settings: LibrarySourceBlock=|
      | simulink/Logic and Bit
      | Operations/Compare
      | To Constant
      mask TypeOptions relop: == | ~= | < | <= | >= | >
      mask TypeOptions OutDataTypeStr: Simulink:masks:uint8 | Simulink:masks:boolean
      mask Callback ZeroCross: sl('zeroCrossEnable', gcbh);
      mask Display: disp(str)
  Constant : Constant  Value=k_gain
  Constant1 : Constant  Value=0.06  SampleTime=1/freq_mag
  Discrete Derivative1 : Subsystem  mask(Discrete Derivative){gainval=1.0, ICPrevScaledInput=0, InputProcessing=Elements as channels (sample based), OutMin=[], OutMax=[], OutDataTypeStr=Inherit: Inherit via internal rule, OutputDataTypeScalingMode=Inherit via internal rule, OutDataType=fixdt(1, 16), OutScaling=2^-10, LockScale=off, RndMeth=Floor, DoSatur=off}
      mask prompts: gainval "Simulink:masks:GainValue_MP"; ICPrevScaledInput "Simulink:masks:InitialConditionForPreviousWeightedInputKuTs_MP"; InputProcessing "Simulink:masks:InputProcessing_MP"; OutMin "Simulink:masks:OutputMinimum_MP"; OutMax "Simulink:masks:OutputMaximum_MP"; OutDataTypeStr "Simulink:masks:OutputDataType_MP"; OutputDataTypeScalingMode "Simulink:masks:OutputDataTypeMode_MP"; OutDataType "Simulink:masks:OutputDataTypeegFixdt116Fixdtsingle_MP"; OutScaling "Simulink:masks:OutputScalingSlopeEg29OrSlopeBias_MP"; LockScale "Simulink:masks:LockOutputDataTypeAgainstFxpTools_MP"; RndMeth "Simulink:masks:IntegerRoundingMode_MP"; DoSatur "Simulink:masks:SaturateToMaxOrMinWhenOverflowsOccur_MP"
      mask help: Simulink:masks:DiscreteDerivative_MD
      mask init:
      | blkH = gcbh;
      | blkName = getfullname(blkH);
      | 
      | if (gainval == 0.0)
      |     %avoid divide by zero warning
      |     inverseGainval = inf;
      | else
      |     inverseGainval = 1.0/double(gainval);
      | end
      | 
      | if isequal(OutDataTypeStr, 'Inherit: Inherit via internal rule')
      |     diffDT   = 'Inherit: Inherit via back propagation';
      |     tsampDT  = 'Inherit: Inherit via internal rule';
      |     tsampImp = 'Offline Scaling Adjustment';
      | else    
      |     diffDT   = OutDataTypeStr;
      |     tsampDT  = 'Inherit: Inherit via back propagation';
      |     tsampImp = 'Online Calculations';
      | end
      | 
      | if ~strcmp(get_param(bdroot(blkH),'SimulationStatus'), 'running')
      |     set_param([blkName,'/Diff'], ...
      |               'RndMeth',RndMeth, ...
      | 	          'DoSatur',DoSatur);
      |     set_param([blkName,'/TSamp'], ...
      |               'OutDataTypeStr',tsampDT, ...
      |               'RndMeth',RndMeth, ...
      |               'DoSatur',DoSatur, ...
      |               'TsampMathImp',tsampImp);
      | end
      | 
      | set_param([blkName,'/UD'], ...
      | 	'InputProcessing',InputProcessing);
      settings: LibrarySourceBlock=simulink/Discrete/Discrete Derivative
      mask TypeOptions InputProcessing: Simulink:masks:ColumnsAsChannelsFrameBased | Simulink:masks:ElementsAsChannelsSampleBased
      mask Callback OutDataTypeStr: fixptdialog(gcbh)
      mask TypeOptions OutputDataTypeScalingMode: double | single | int8 | uint8 | int16 | uint16 | int32 | uint32 | Specify via dialog | Inherit via internal rule | Inherit via back propagation
      mask Callback OutputDataTypeScalingMode: fixptdialog(gcbh)
      mask Callback OutDataType: fixptdialog(gcbh)
      mask TypeOptions RndMeth: Simulink:masks:Ceiling | Simulink:masks:Convergent | Simulink:masks:Floor | Simulink:masks:Nearest | Simulink:masks:Round | Simulink:masks:Simplest | Simulink:masks:Zero
      mask Display: text(0.5, 0.5, 'K (z-1)', 'horizontalAlignment', 'center', 'verticalAlignment', 'bottom');text(0.5, 0.5, 'Ts z', 'horizontalAlignment', 'center', 'verticalAlignment', 'top');plot([0.3 0.7],[0.5 0.5]);
  Discrete Varying Lowpass1 : Subsystem  mask(Discrete Varying Lowpass){N=1, w0=0, Ts=1/freq_mag}
      mask prompts: N "Control:simulink:VaryingLowpassLabel1"; w0 "Control:simulink:VaryingLowpassLabel2"; Ts "Control:simulink:VaryingLowpassLabel3"
      mask help: Control:simulink:VaryingLowpass2
      mask init: same as complete_model_sim_nolib/ Actuators/Discrete Varying Lowpass
      settings: LibrarySourceBlock=cstblocks/Linear Parameter Varying/Discrete Varying Lowpass
      mask Help: eval('helpview(''control'',''VaryingLowpassDT'');')
      mask DialogControl N Prompt: Filter order:
      mask DialogControl w0 Prompt: Pre-warping frequency w0 (rad/s):
      mask DialogControl Ts Prompt: Sample time Ts:
      mask Display:
      | image('lowpass_dt.png',[0.1 0 0.8 1]);
      | port_label('input', 2, 'freq');
  Divide : Product  Inputs=*/
  Dot Product : DotProduct  OutDataTypeStr=Inherit: Inherit via internal rule
  Dot Product1 : DotProduct  OutDataTypeStr=Inherit: Inherit via internal rule
  Gain : Gain  Gain=-1
  Normalize Vector : Subsystem  mask(Normalize Vector){maxzero=0}
      mask prompts: maxzero "Maximum modulus to treat vector as zero:"
      mask help:
      | Normalize a vector.
      | Output is the unit vector parallel to the input vector. Input can be vector of any size.
      | If the modulus of the input is lower or equal than specified, the output is set to zeros(size(u)).
      settings: LibrarySourceBlock=vrlib/Utilities/Normalize Vector
      mask Help: helpview(vrmfunc('FnHelpTopic'), 'vr_normalizevector');
      mask Display: disp('Normalize')
  OR : Logic  Operator=OR  IconShape=distinctive  AllPortsSameDT=off  OutDataTypeStr=boolean
  Product : Product
  Scope{,1..4} (5 alike) : Scope
  Sqrt : Sqrt
  Sqrt1 : Sqrt
  Vector Concatenate1 : Concatenate  NumInputs=3
  Zero : Constant  Value=0  OutDataTypeStr=Inherit: Inherit via back propagation
  cmd : Outport
  flag : Outport  Port=2
  wires:
  Dot Product/1 -> Sqrt/1
  Constant/1 -> Gain/1  "k"
  Divide/1 -> Scope4/1, Product/1
  Product/1 -> Vector Concatenate1/1, Scope/1  "m"
  Sqrt/1 -> Divide/2  "|B_m|"
  Gain/1 -> Divide/1
  Normalize Vector/1(Out1) -> Discrete Derivative1/1(U)
  B_m/1 -> Dot Product/2, Normalize Vector/1(In1), Dot Product/1
  Discrete Derivative1/1(Y) -> Discrete Varying Lowpass1/1(u), Scope3/1
  Sqrt1/1 -> Compare To Constant/1(u), Scope2/1
  Dot Product1/1 -> Sqrt1/1
  OR/1 -> flag/1
  Compare To Constant/1(y) -> OR/1
  Compare To Constant1/1(y) -> OR/2
  Clock/1 -> Compare To Constant1/1(u)
  Constant1/1 -> Discrete Varying Lowpass1/2(frequency)
  Discrete Varying Lowpass1/1(y) -> Scope1/1, Dot Product1/2, Dot Product1/1, Product/2
  Vector Concatenate1/1 -> cmd/1
  Zero/1 -> Vector Concatenate1/3, Vector Concatenate1/2

== system complete_model_sim_nolib/Control/Slew Maneuver ==
  Abn_sens : Inport
  Aln : Inport  Port=2
  B_m : Inport  Port=3
  Enable : EnablePort
  Control Logic : Subsystem
  Gain : Gain  Gain=-0.6
  Gain2 : Gain  Gain=-0.01
  Matrix Multiply : Product  Multiplication=Matrix(*)
  Scope : Scope
  Sum : Sum
  Transpose : Math  Operator=transpose
  compute alphadots : Subsystem
  compute alphas : Subsystem
  cmd : Outport
  wires:
  Aln/1 -> Transpose/1
  Transpose/1 -> Matrix Multiply/2
  Abn_sens/1 -> Matrix Multiply/1, compute alphadots/1(Abn)
  Matrix Multiply/1 -> compute alphas/1(Abl), compute alphadots/2(Abl)
  compute alphadots/1(Alphadots) -> Gain/1
  compute alphas/1(estimated state) -> Scope/1, Gain2/1
  Gain/1 -> Sum/1
  Gain2/1 -> Sum/2
  B_m/1 -> Control Logic/2(B_m)
  Sum/1 -> Control Logic/1(u)
  Control Logic/1(cmd) -> cmd/1

== system complete_model_sim_nolib/Disturbances/Magnetic Torque  ==
  rn : Inport
  Abn : Inport  Port=2
  Constant3 : Constant  Value=jb
  Cross Product : matrix_library/Cross Product
  Matrix Multiply1 : Product  Multiplication=Matrix(*)
  Scope : Scope
  To Workspace : ToWorkspace  VariableName=mag_tor  SampleTime=-1
  compute Bn : Subsystem
  M_mag : Outport
  Bb : Outport  Port=2
  wires:
  Constant3/1 -> Cross Product/1
  Matrix Multiply1/1 -> Cross Product/2, Bb/1
  Cross Product/1 -> To Workspace/1, M_mag/1
  compute Bn/1(Bn) -> Matrix Multiply1/2, Scope/1
  rn/1 -> compute Bn/1(rN)
  Abn/1 -> Matrix Multiply1/1

== system complete_model_sim_nolib/Disturbances/gravity torque ==
  c : Inport
  rnorm : Inport  Port=2
  Constant : Constant  Value=mu
  Constant1 : Constant  Value=I
  Constant3 : Constant  Value=3
  Cross Product : matrix_library/Cross Product
  Divide : Product  Inputs=**/
  Gain : Gain  Gain=-1
  Matrix Multiply : Product  Multiplication=Matrix(*)
  Power : Math  Operator=pow
  Product : Product
  Mg : Outport
  wires:
  Constant1/1 -> Matrix Multiply/1
  c/1 -> Matrix Multiply/2, Cross Product/2
  Matrix Multiply/1 -> Cross Product/1
  Constant3/1 -> Power/2, Divide/2
  Power/1 -> Divide/3
  Constant/1 -> Divide/1
  Divide/1 -> Gain/1
  Gain/1 -> Product/2
  Cross Product/1 -> Product/1
  Product/1 -> Mg/1
  rnorm/1 -> Power/1

== system complete_model_sim_nolib/Disturbances/norm ==
  rn : Inport
  Dot Product : DotProduct  OutDataTypeStr=Inherit: Inherit via internal rule
  Sqrt : Sqrt
  rnorm : Outport
  wires:
  rn/1 -> Dot Product/1, Dot Product/2
  Dot Product/1 -> Sqrt/1
  Sqrt/1 -> rnorm/1

== system complete_model_sim_nolib/Dynamics/Cross Product ==
  note: Cross product of two 3x1 vectors a=[a1 a2 a3], b=[b1 b2 b3]:
      | y = a x b = (a2b3-a3b2)i + (a3b1-a1b3)j + (a1b2-a2b1)k
  a : Inport
  b : Inport  Port=2
  Element Product : Product  RndMeth=Simplest
  Selector2 : Selector  InputPortWidth=6  IndexOptions=Index vector (dialog)  Indices=[1 2 3]  OutputSizes=1
  Selector3 : Selector  InputPortWidth=6  IndexOptions=Index vector (dialog)  Indices=[4 5 6]  OutputSizes=1
  Sum : Sum  Inputs=+|-  RndMeth=Simplest
  a elements : Selector  InputPortWidth=3  IndexOptions=Index vector (dialog)  Indices=[2 3 1 3 1 2]  OutputSizes=1
  b elements : Selector  InputPortWidth=3  IndexOptions=Index vector (dialog)  Indices=[3 1 2 2 3 1]  OutputSizes=1
  y : Outport
  wires:
  Selector3/1 -> Sum/2
  Selector2/1 -> Sum/1
  Element Product/1 -> Selector2/1, Selector3/1
  b/1 -> b elements/1
  b elements/1 -> Element Product/2
  a elements/1 -> Element Product/1
  Sum/1 -> y/1
  a/1 -> a elements/1

== system complete_model_sim_nolib/Horizon Sensor/EH sensor modeling ==
  rb : Inport
  Cross Product : Subsystem  mask(CrossProduct){}
      mask help: Simulink:masks:MatLibCrossProduct_MD
      settings: LibrarySourceBlock=|
      | simulink/Matrix
      | Operations/Cross Product
      mask Display: disp('cross')
  Normalize Vector : Subsystem  mask(Normalize Vector){maxzero=0}
      mask prompts: maxzero "Maximum modulus to treat vector as zero:"
      mask help:
      | Normalize a vector.
      | Output is the unit vector parallel to the input vector. Input can be vector of any size.
      | If the modulus of the input is lower or equal than specified, the output is set to zeros(size(u)).
      settings: LibrarySourceBlock=vrlib/Utilities/Normalize Vector
      mask Help: helpview(vrmfunc('FnHelpTopic'), 'vr_normalizevector');
      mask Display: disp('Normalize')
  Product : Product
  Sum2 : Sum
  Uniform Random Number : UniformRandomNumber  SampleTime=1/30
  Uniform Random Number1 : UniformRandomNumber  SampleTime=1/30
  Uniform Random Number2 : UniformRandomNumber  SampleTime=1/30
  Uniform Random Number3 : UniformRandomNumber  Minimum=0  Maximum=tan(deg2rad(0.1))*0.1  SampleTime=1/30
  Vector Concatenate : Concatenate  NumInputs=3
  Zero-Order Hold : ZeroOrderHold  SampleTime=1/freq_earth
  q : Outport
  wires:
  Product/1 -> Sum2/1
  Uniform Random Number3/1 -> Product/1
  Uniform Random Number1/1 -> Vector Concatenate/2
  Uniform Random Number2/1 -> Vector Concatenate/3
  Normalize Vector/1(Out1) -> Product/2
  Uniform Random Number/1 -> Vector Concatenate/1
  Zero-Order Hold/1 -> Cross Product/2(b), Sum2/2  "R_B"
  Vector Concatenate/1 -> Cross Product/1(a)
  Cross Product/1(y) -> Normalize Vector/1(In1)
  Sum2/1 -> q/1  "q"
  rb/1 -> Zero-Order Hold/1

== system complete_model_sim_nolib/Horizon Sensor/FOV CHECK ==
  rb : Inport
  Acos : Trigonometry  Operator=acos
  Dot Product : DotProduct  OutDataTypeStr=Inherit: Inherit via internal rule
  FOV angle : Constant  Value=FOV_earth
  Gain : Gain  Gain=-1
  Less Than : RelationalOperator  Operator=<  OutDataTypeStr=boolean  RndMeth=Simplest  InputSameDT=off
  optical axis : Constant  Value=[-1;0;0]
  b : Outport
  wires:
  optical axis/1 -> Dot Product/1
  Dot Product/1 -> Acos/1
  FOV angle/1 -> Less Than/2
  Acos/1 -> Less Than/1
  Less Than/1 -> b/1
  Gain/1 -> Dot Product/2
  rb/1 -> Gain/1

== system complete_model_sim_nolib/Kinematics/Kinematics 312 ==
  w : Inport
  Enable : EnablePort  StatesWhenEnabling=reset
  A - s_312 : Subsystem
  Euler angles : Subsystem
  IC : InitialCondition  Value=s0
  s_312 - A : Subsystem
  s_313 - A : Subsystem
  A : Outport
  wires:
  s_312 - A/1(A) -> A/1  "A"
  Euler angles/1(s) -> s_312 - A/1(s)  "s"
  w/1 -> Euler angles/1(w)
  IC/1 -> Euler angles/2(s0)
  A - s_312/1(s) -> IC/1
  s_313 - A/1(A) -> A - s_312/1(A)
  [s_313] -> s_313 - A/1(s)

== system complete_model_sim_nolib/Kinematics/Kinematics 313 ==
  w : Inport
  Enable : EnablePort  StatesWhenEnabling=reset
  A - s_313 : Subsystem
  Euler angles : Subsystem
  s_312 - A : Subsystem
  s_313 - A : Subsystem
  A : Outport
  wires:
  w/1 -> Euler angles/1(w)
  Euler angles/1(s) -> s_313 - A/1(s)
  s_313 - A/1(A) -> A/1
  A - s_313/1(s) -> Euler angles/2(s0)
  s_312 - A/1(A) -> A - s_313/1(A)
  [s_312] -> s_312 - A/1(s)
